simulink model "Steering_Plant_Model_Pi"  (R2022b)
settings: Solver=FixedStepAuto  StartTime=0.0  StopTime=56  RelTol=1e-3  EnableMultiTasking=on
libraries: canmsglib x2, raspberrypiCommlib x2, simulink x2
settings Model: Creator=david  LastModifiedBy=david
settings SolverCC: PositivePriorityOrder=on
settings OptimizationCC: EnhancedBackFolding=on  PassReuseOutputArgsAs=Individual arguments  ZeroExternalMemoryAtStartup=off  ZeroInternalMemoryAtStartup=off  MaxStackSize=64  OptimizeBlockOrder=speed  DifferentSizesBufferReuse=on  OptimizationCustomize=off  EfficientTunableParamExpr=on
settings DebuggingCC: ParameterTunabilityLossMsg=error
settings HardwareCC: ProdBitPerPointer=32  ProdBitPerSizeT=32  ProdBitPerPtrDiffT=32  ProdLargestAtomicInteger=Long  ProdLargestAtomicFloat=Double  ProdWordSize=32  ProdLongLongMode=on  ProdHWDeviceType=ARM Compatible->ARM Cortex
settings RTWCC: Description=Embedded Coder  SystemTargetFile=ert.tlc  HardwareBoard=Raspberry Pi  TLCOptions="-aInlineSetEventsForThisBaseRateFcn=TLC_FALSE -aSuppressMultiTaskScheduler=TLC_FALSE  -aRateBasedStepFcn=0"  TemplateMakefile=ert_default_tmf  Toolchain=GNU GCC Embedded Linux  BuildConfiguration=Faster Runs
settings CodeAppCC: ForceParamTrailComments=on  IgnoreCustomStorageClasses=off  OperatorAnnotations=on  SimulinkDataObjDesc=on  SFDataObjDesc=on  InsertBlockDesc=on
settings ERTTargetCC: SupportContinuousTime=on  SupportVariableSizeSignals=on  ExtModeTransport=2  ExtModeStaticAlloc=on  ExtModeMexFile=ext_xcp  ExtModeIntrfLevel=Level2 - Open

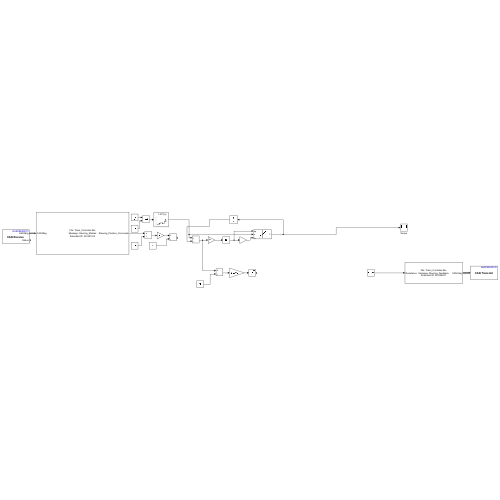
[thumbnail: Simulink's stored preview of the top-level diagram]
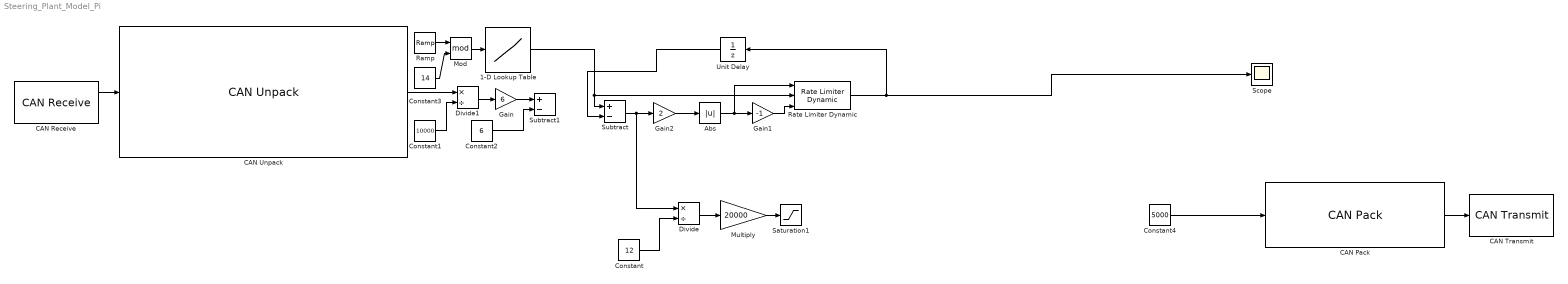
== system Steering_Plant_Model_Pi ==
  1-D Lookup Table : Lookup_n-D  NumberOfTableDimensions=1  LookupTableObject=''  BreakpointsForDimension1=[0,2,4,6,8,10,12,14]  BreakpointsForDimension1FirstPoint=10  BreakpointsForDimension2FirstPoint=10  BreakpointsForDimension1Spacing=12  BreakpointsForDimension2Spacing=12  IndexSearchMethod=Evenly spaced points  Table=[0,6,12,0,6,6,6,12]  InterpMethod=Flat  DiagnosticForOutOfRangeInput=Error  InternalRulePriority=Speed  RndMeth=Simplest
  Abs : Abs  SaturateOnIntegerOverflow=off
  CAN Pack : canmsglib/CAN Pack  CANdbFile=C:\Git\2023_Tractor_Plant_Models\23_Trans\Trans_Controller.dbc  MsgList=Steering_Feedback  MsgName=Steering_Feedback  MsgIDType=Extended (29-bit identifier)  MsgIdentifier=201524227  MsgLength=8  Remote=off  ApplyMinMax=off  BusOutput=on  SignalInfo={'Resistance','0','16','LE','unsigned','Standard','0','1','10000','-10000','10000'}
      settings: LibrarySourceBlock=embeddedtargetslib/Host Communication/CAN Pack  DataFormat=CANdb specified signals
  CAN Receive : raspberrypiCommlib/CAN Receive  DeviceID=can0  SetupCAN=off  TypeofCAN=Real  OutputDataType=CAN Msg  IdentifierType=Standard (11-bit identifier)  MessageId=100  MsgLength=8  SampleTime=-1  OutputError=off  OutputRemote=off  SimulateUsing=Code generation
  CAN Transmit : raspberrypiCommlib/CAN Transmit  DeviceID=can0  SetupCAN=on  TypeofCAN=Real  InputDataType=CAN Msg  BlockingMode_=off  BlockTimeout_=1  OutputStatus=off  IdentifierType=Standard (11-bit identifier)  MessageId=100  MsgLength=8  RemoteFrame=off  SimulateUsing=Code generation
  CAN Unpack : canmsglib/CAN Unpack  CANdbFile=C:\Git\2023_Tractor_Plant_Models\23_Trans\Trans_Controller.dbc  MsgList=Steering_Module  MsgName=Steering_Module  MsgIDType=Extended (29-bit identifier)  MsgIdentifier=201457412  MsgLength=8  SignalInfo={'Steering_Position_Command','0','16','LE','unsigned','Standard','0','1','10000','-10000','10000'}  IDPort=off  TimestampPort=off  ErrorPort=off  RemotePort=off  LengthPort=off  StatusPort=off  ApplyMinMax=off
      settings: LibrarySourceBlock=embeddedtargetslib/Host Communication/CAN Unpack  DataFormat=CANdb specified signals
  Constant : Constant  Value=12
  Constant1 : Constant  Value=10000
  Constant2 : Constant  Value=6
  Constant3 : Constant  Value=14
  Constant4 : Constant  Value=5000
  Divide : Product  Inputs=*/
  Divide1 : Product  Inputs=*/
  Gain : Gain  Gain=6
  Gain1 : Gain  Gain=-1
  Gain2 : Gain  Gain=2
  Mod : Math  Operator=mod
  Multiply : Gain  Gain=20000
  Ramp : simulink/Sources/Ramp  slope=1  start=0  InitialOutput=0
  Rate Limiter Dynamic : simulink/Discontinuities/Rate Limiter Dynamic
  Saturation1 : Saturate  UpperLimit=10000  LowerLimit=-10000
  Scope : Scope
  Subtract : Sum  Inputs=+-
  Subtract1 : Sum  Inputs=+-
  Unit Delay : UnitDelay  SampleTime=-1  HasFrameUpgradeWarning=on
  wires:
  CAN Receive/1 -> CAN Unpack/1
  Gain/1 -> Subtract1/1
  CAN Unpack/1 -> Divide1/1
  Multiply/1 -> Saturation1/1
  Constant/1 -> Divide/2
  Constant2/1 -> Subtract1/2
  Divide/1 -> Multiply/1
  Unit Delay/1 -> Subtract/2
  Subtract/1 -> Gain2/1, Divide/1
  Constant1/1 -> Divide1/2
  Divide1/1 -> Gain/1
  CAN Pack/1 -> CAN Transmit/1
  Rate Limiter Dynamic/1 -> Unit Delay/1, Scope/1
  1-D Lookup Table/1 -> Rate Limiter Dynamic/2, Subtract/1
  Abs/1 -> Gain1/1, Rate Limiter Dynamic/1
  Gain1/1 -> Rate Limiter Dynamic/3
  Gain2/1 -> Abs/1
  Mod/1 -> 1-D Lookup Table/1
  Ramp/1 -> Mod/1
  Constant3/1 -> Mod/2
  Constant4/1 -> CAN Pack/1
